simulink subsystem "DKE_detumbling"  (R2021a)
settings: Solver=VariableStepAuto  StartTime=0.0  StopTime=10.0  RelTol=1e-3
libraries: aerolibutil x1
settings Model: Creator=Laura  LastModifiedBy=Laura

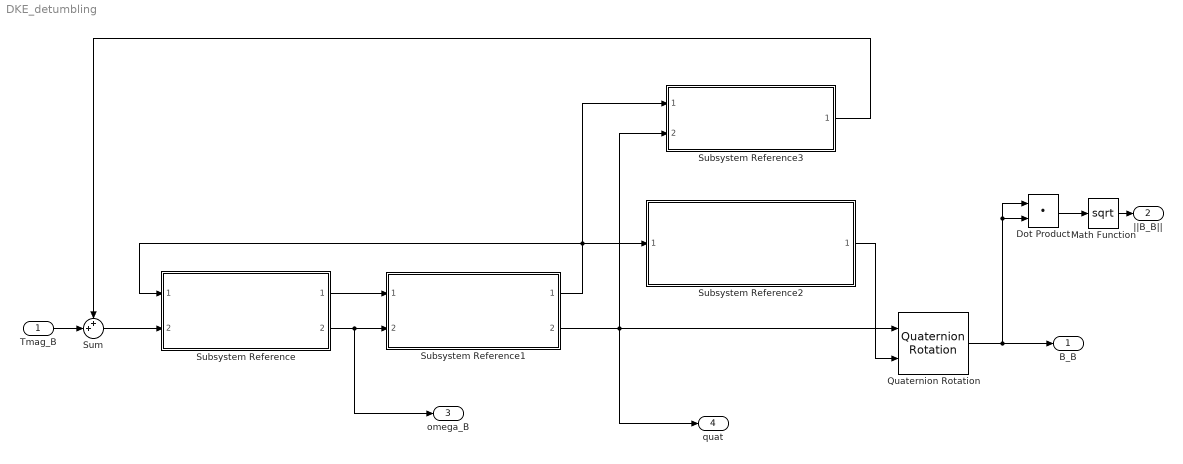
== system DKE_detumbling ==
  Tmag_B : Inport
  Dot Product : DotProduct  InputSameDT=on  OutDataTypeStr=Inherit: Inherit via internal rule
  Math Function : Math  Operator=sqrt  SignedPower=on  SaturateOnIntegerOverflow=on
  Quaternion Rotation : aerolibutil/Quaternion Rotation
  Subsystem Reference : Subsystem  ReferencedSubsystem=Dynamics
  Subsystem Reference1 : Subsystem  ReferencedSubsystem=Kinematics
  Subsystem Reference2 : Subsystem  ReferencedSubsystem=MagnetoField
  Subsystem Reference3 : Subsystem  ReferencedSubsystem=GravityTorque
  Sum : Sum  Inputs=++|
  B_B : Outport
  ||B_B|| : Outport  Port=2
  omega_B : Outport  Port=3
  quat : Outport  Port=4
  wires:
  Subsystem Reference/1 -> Subsystem Reference1/1
  Subsystem Reference/2 -> omega_B/1, Subsystem Reference1/2
  Quaternion Rotation/1 -> B_B/1, Dot Product/2, Dot Product/1
  Subsystem Reference2/1 -> Quaternion Rotation/2
  Math Function/1 -> ||B_B||/1
  Dot Product/1 -> Math Function/1
  Subsystem Reference1/2 -> quat/1, Quaternion Rotation/1, Subsystem Reference3/2
  Subsystem Reference1/1 -> Subsystem Reference2/1, Subsystem Reference/1, Subsystem Reference3/1
  Sum/1 -> Subsystem Reference/2
  Tmag_B/1 -> Sum/2
  Subsystem Reference3/1 -> Sum/1
